simulink model "D2C_boucle_vitesse_acompleter"  (R2013a)
settings: Solver=ode45  StartTime=0.0  StopTime=6  FixedStep=0.003  RelTol=1e-3
settings Model: Creator=Propriétaire  LastModifiedBy=Administrateur
settings DataIOCC: SignalLoggingSaveFormat=ModelDataLogs
settings OptimizationCC: ExpressionDepthLimit=2147483647
settings DebuggingCC: FcnCallInpInsideContextMsg=UseLocalSettings
settings GRTTargetCC: CombineOutputUpdateFcns=off  GRTInterface=on

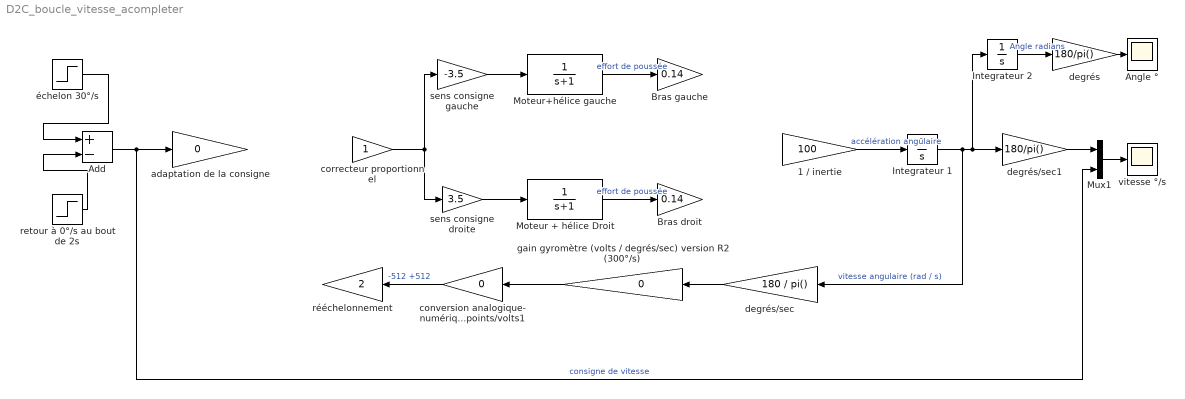
== system D2C_boucle_vitesse_acompleter ==
  1 / inertie : Gain  Gain=100
  Add : Sum  Inputs=+-
  Angle ° : Scope
      settings: YMin=-1  YMax=10
  Bras droit : Gain  Gain=0.14
  Bras gauche : Gain  Gain=0.14
  Integrateur 1 : Integrator
  Integrateur 2 : Integrator
  Moteur + hélice Droit : TransferFcn  Denominator=[1 1]
  Moteur+hélice gauche : TransferFcn  Denominator=[1 1]
  Mux1 : Mux  Inputs=2
  adaptation de la consigne : Gain  Gain=0
  conversion analogique- numérique points/volts1 : Gain  Gain=0
  correcteur proportionnel : Gain
  degrés : Gain  Gain=180/pi()
  degrés/sec : Gain  Gain=180 / pi()
  degrés/sec1 : Gain  Gain=180/pi()
  gain gyromètre (volts / degrés/sec) version R2 (300°/s) : Gain  Gain=0
  retour à 0°/s au bout de 2s : Step  Time=2  After=30  SampleTime=0
  rééchelonnement : Gain  Gain=2
  sens consigne droite : Gain  Gain=3.5
  sens consigne gauche : Gain  Gain=-3.5
  vitesse °/s : Scope
      settings: YMin=-1  YMax=10  SaveName=ScopeData4
  échelon 30°/s : Step  Time=0  After=30  SampleTime=0
  wires:
  Moteur+hélice gauche/1 -> Bras gauche/1  "effort de poussée"
  Moteur + hélice Droit/1 -> Bras droit/1  "effort de poussée"
  gain gyromètre (volts / degrés/sec) version R2 (300°/s)/1 -> conversion analogique- numérique points/volts1/1
  Integrateur 2/1 -> degrés/1  "Angle radians"
  1 / inertie/1 -> Integrateur 1/1  "accélération angulaire"
  Integrateur 1/1 -> Integrateur 2/1, degrés/sec1/1, degrés/sec/1  "vitesse angulaire (rad / s)"
  degrés/sec/1 -> gain gyromètre (volts / degrés/sec) version R2 (300°/s)/1
  degrés/1 -> Angle °/1
  Add/1 -> Mux1/2, adaptation de la consigne/1  "consigne de vitesse"
  degrés/sec1/1 -> Mux1/1
  conversion analogique- numérique points/volts1/1 -> rééchelonnement/1  "-512 +512"
  Mux1/1 -> vitesse °/s/1
  sens consigne droite/1 -> Moteur + hélice Droit/1
  sens consigne gauche/1 -> Moteur+hélice gauche/1
  échelon 30°/s/1 -> Add/1
  retour à 0°/s au bout de 2s/1 -> Add/2
  correcteur proportionnel/1 -> sens consigne gauche/1, sens consigne droite/1
